simulink model "P5PIDModel"  (R2015b)
settings: Solver=FixedStepAuto  StartTime=0.0  StopTime=inf  FixedStep=1  RelTol=1e-1  AbsTol=1e-1
undefined symbols (not defined in the file or in its folder): D, PI
libraries: fuzblock x2
settings Model: Creator=Pepe  LastModifiedBy=Pepe
settings SolverCC: ConsecutiveZCsStepRelTol=10*128*eps / 100
settings OptimizationCC: BlockReduction=off  BooleanDataType=off  InitFltsAndDblsToZero=on
settings HardwareCC: ProdBitPerPointer=32  ProdWordSize=32  ProdHWDeviceType=Intel->x86-32 (Windows32)

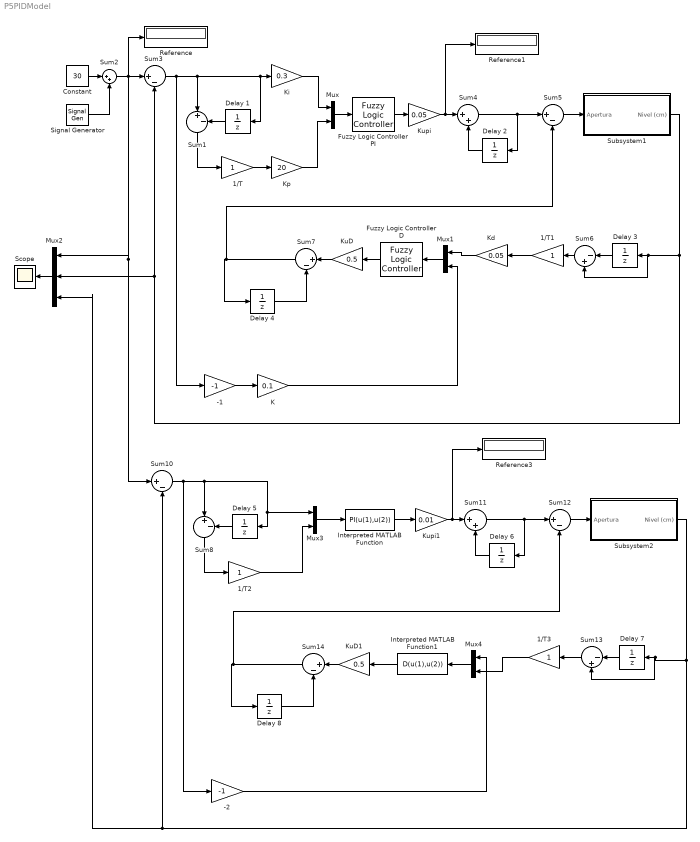
== system P5PIDModel ==
  -1 : Gain  Gain=-1  SaturateOnIntegerOverflow=on  OutDataTypeStr=Inherit: Same as input  ParamDataTypeStr=Inherit: Same as input
  -2 : Gain  Gain=-1  SaturateOnIntegerOverflow=on  OutDataTypeStr=Inherit: Same as input  ParamDataTypeStr=Inherit: Same as input
  1/T{,1..3} (4 alike) : Gain  SaturateOnIntegerOverflow=on  OutDataTypeStr=Inherit: Same as input  ParamDataTypeStr=Inherit: Same as input
  Constant : Constant  Value=30
  Delay {1..8} (8 alike) : UnitDelay
  Fuzzy Logic Controller D : fuzblock/Fuzzy Logic  Controller  fis=DFuzzy
  Fuzzy Logic Controller PI : fuzblock/Fuzzy Logic  Controller  fis=PIFuzzy
  Interpreted MATLAB Function : MATLABFcn  MATLABFcn=PI(u(1),u(2))
  Interpreted MATLAB Function1 : MATLABFcn  MATLABFcn=D(u(1),u(2))
  K : Gain  Gain=0.1  SaturateOnIntegerOverflow=on  OutDataTypeStr=Inherit: Same as input  ParamDataTypeStr=Inherit: Same as input
  Kd : Gain  Gain=0.05  SaturateOnIntegerOverflow=on  OutDataTypeStr=Inherit: Same as input  ParamDataTypeStr=Inherit: Same as input
  Ki : Gain  Gain=0.3  SaturateOnIntegerOverflow=on  OutDataTypeStr=Inherit: Same as input  ParamDataTypeStr=Inherit: Same as input
  Kp : Gain  Gain=20  SaturateOnIntegerOverflow=on  OutDataTypeStr=Inherit: Same as input  ParamDataTypeStr=Inherit: Same as input
  KuD : Gain  Gain=0.5  SaturateOnIntegerOverflow=on  OutDataTypeStr=Inherit: Same as input  ParamDataTypeStr=Inherit: Same as input
  KuD1 : Gain  Gain=0.5  SaturateOnIntegerOverflow=on  OutDataTypeStr=Inherit: Same as input  ParamDataTypeStr=Inherit: Same as input
  Kupi : Gain  Gain=0.05  SaturateOnIntegerOverflow=on  OutDataTypeStr=Inherit: Same as input  ParamDataTypeStr=Inherit: Same as input
  Kupi1 : Gain  Gain=0.01  SaturateOnIntegerOverflow=on  OutDataTypeStr=Inherit: Same as input  ParamDataTypeStr=Inherit: Same as input
  Mux{,1,3..4} (4 alike) : Mux  Inputs=2
  Mux2 : Mux  Inputs=3
  Reference : Display
  Reference1 : Display
  Reference3 : Display
  Scope : Scope
  Signal Generator : SignalGenerator  WaveForm=square  Amplitude=10  Frequency=0.0001
  Subsystem1 : Subsystem
  Subsystem2 : Subsystem
  Sum{1,3,5,7..8,10,12,14} (8 alike) : Sum  Inputs=|+-  SaturateOnIntegerOverflow=on  InputSameDT=on  OutDataTypeStr=Inherit: Same as first input
  Sum11 : Sum  Inputs=|++  SaturateOnIntegerOverflow=on  InputSameDT=on  OutDataTypeStr=Inherit: Same as first input
  Sum13 : Sum  Inputs=|-+  SaturateOnIntegerOverflow=on  InputSameDT=on  OutDataTypeStr=Inherit: Same as first input
  Sum2 : Sum  Inputs=|++  SaturateOnIntegerOverflow=on  InputSameDT=on  OutDataTypeStr=Inherit: Same as first input
  Sum4 : Sum  Inputs=|++  SaturateOnIntegerOverflow=on  InputSameDT=on  OutDataTypeStr=Inherit: Same as first input
  Sum6 : Sum  Inputs=|-+  SaturateOnIntegerOverflow=on  InputSameDT=on  OutDataTypeStr=Inherit: Same as first input
  wires:
  Constant/1 -> Sum2/1
  Signal Generator/1 -> Sum2/2
  Sum2/1 -> Sum10/1, Mux2/1, Sum3/1, Reference/1
  Sum3/1 -> -1/1, Sum1/1, Delay 1/1, Ki/1
  Delay 1/1 -> Sum1/2
  1/T/1 -> Kp/1
  Kp/1 -> Mux/2
  Ki/1 -> Mux/1
  Mux/1 -> Fuzzy Logic Controller PI/1
  Fuzzy Logic Controller PI/1 -> Kupi/1
  Kupi/1 -> Reference1/1, Sum4/1
  Delay 2/1 -> Sum4/2
  Sum4/1 -> Sum5/1, Delay 2/1
  Sum5/1 -> Subsystem1/1(Apertura)
  Subsystem1/1(Nivel (cm)) -> Sum6/2, Delay 3/1, Sum3/2, Mux2/2
  Delay 3/1 -> Sum6/1
  Sum6/1 -> 1/T1/1
  Mux1/1 -> Fuzzy Logic Controller D/1
  Kd/1 -> Mux1/1
  -1/1 -> K/1
  K/1 -> Mux1/2
  Fuzzy Logic Controller D/1 -> KuD/1
  KuD/1 -> Sum7/1
  Delay 4/1 -> Sum7/2
  Sum7/1 -> Sum5/2, Delay 4/1
  Mux2/1 -> Scope/1
  Delay 5/1 -> Sum8/2
  Sum8/1 -> 1/T2/1
  1/T2/1 -> Mux3/2
  Sum10/1 -> -2/1, Sum8/1, Mux3/1, Delay 5/1
  Interpreted MATLAB Function/1 -> Kupi1/1
  Kupi1/1 -> Reference3/1, Sum11/1
  Delay 6/1 -> Sum11/2
  Sum11/1 -> Sum12/1, Delay 6/1
  Sum12/1 -> Subsystem2/1(Apertura)
  Subsystem2/1(Nivel (cm)) -> Sum13/2, Delay 7/1, Mux2/3, Sum10/2
  Delay 7/1 -> Sum13/1
  Sum13/1 -> 1/T3/1
  KuD1/1 -> Sum14/1
  Delay 8/1 -> Sum14/2
  Sum14/1 -> Sum12/2, Delay 8/1
  Mux3/1 -> Interpreted MATLAB Function/1
  Interpreted MATLAB Function1/1 -> KuD1/1
  Mux4/1 -> Interpreted MATLAB Function1/1
  1/T3/1 -> Mux4/2
  -2/1 -> Mux4/1
  Sum1/1 -> 1/T/1
  1/T1/1 -> Kd/1

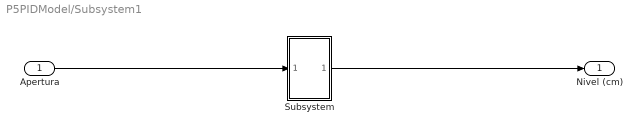
== system P5PIDModel/Subsystem1 ==
  Apertura : Inport
  Subsystem : Subsystem
  Nivel (cm) : Outport
  wires:
  Subsystem/1(Out1) -> Nivel (cm)/1
  Apertura/1 -> Subsystem/1(In1)

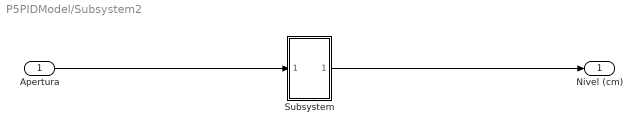
== system P5PIDModel/Subsystem2 ==
  Apertura : Inport
  Subsystem : Subsystem
  Nivel (cm) : Outport
  wires:
  Subsystem/1(Out1) -> Nivel (cm)/1
  Apertura/1 -> Subsystem/1(In1)

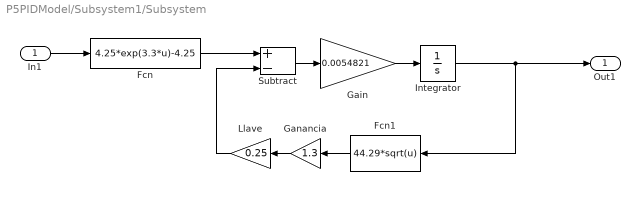
== system P5PIDModel/Subsystem1/Subsystem ==
  In1 : Inport
  Fcn : Fcn  Expr=4.25*exp(3.3*u)-4.25
  Fcn1 : Fcn  Expr=44.29*sqrt(u)
  Gain : Gain  Gain=0.0054821
  Ganancia : Gain  Gain=1.3
  Integrator : Integrator  InitialCondition=15  LimitOutput=on  UpperSaturationLimit=78  LowerSaturationLimit=0
  Llave : Gain  Gain=0.25
  Subtract : Sum  Inputs=+-
  Out1 : Outport
  wires:
  Llave/1 -> Subtract/2
  Fcn1/1 -> Ganancia/1
  Gain/1 -> Integrator/1
  Fcn/1 -> Subtract/1
  Ganancia/1 -> Llave/1
  Subtract/1 -> Gain/1
  In1/1 -> Fcn/1
  Integrator/1 -> Out1/1, Fcn1/1

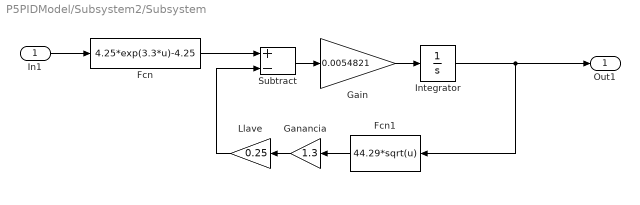
== system P5PIDModel/Subsystem2/Subsystem ==
  In1 : Inport
  Fcn : Fcn  Expr=4.25*exp(3.3*u)-4.25
  Fcn1 : Fcn  Expr=44.29*sqrt(u)
  Gain : Gain  Gain=0.0054821
  Ganancia : Gain  Gain=1.3
  Integrator : Integrator  InitialCondition=15  LimitOutput=on  UpperSaturationLimit=78  LowerSaturationLimit=0
  Llave : Gain  Gain=0.25
  Subtract : Sum  Inputs=+-
  Out1 : Outport
  wires:
  Llave/1 -> Subtract/2
  Fcn1/1 -> Ganancia/1
  Gain/1 -> Integrator/1
  Fcn/1 -> Subtract/1
  Ganancia/1 -> Llave/1
  Subtract/1 -> Gain/1
  In1/1 -> Fcn/1
  Integrator/1 -> Out1/1, Fcn1/1
